simulink model "asbCubeSatACS"  (R2023b)
settings: Solver=FixedStepDiscrete  StartTime=0.0  StopTime=10.0  FixedStep=CubeSatTimeStep  RelTol=1e-3  EnableMultiTasking=on
settings Model: DataDictionary=asbCubeSatModelData.sldd  Creator=The MathWorks, Inc.  LastModifiedBy=bobow
settings SolverCC: AlgebraicLoopSolver=TrustRegion  MaxZcPerStep=1
settings DataIOCC: LimitDataPoints=on  SaveFormat=Array  SaveOutput=off  SignalLogging=off  DSMLogging=off  SaveTime=off  ReturnWorkspaceOutputs=off
settings OptimizationCC: DefaultParameterBehavior=Inlined  OptimizeBlockIOStorage=off  BufferReuse=off  GlobalBufferReuse=off  ExpressionFolding=off  ExpressionDepthLimit=2147483647  LocalBlockOutputs=off  InitFltsAndDblsToZero=on  LifeSpan=inf  OptimizeDataStoreBuffers=off  BusAssignmentInplaceUpdate=off
settings DebuggingCC: ArtificialAlgebraicLoopMsg=none  SolverPrmCheckMsg=warning  FcnCallInpInsideContextMsg=warning  UnconnectedInputMsg=warning  UnconnectedOutputMsg=warning  UnconnectedLineMsg=warning  StateNameClashWarn=warning  PregeneratedLibrarySubsystemCodeDiagnostic=none  SFUnexpectedBacktrackingDiag=warning  SFNoUnconditionalDefaultTransitionDiag=warning  SFExecutionAtInitializationDiag=none  ArithmeticOperatorsInVariantConditions=warning
settings HardwareCC: ProdBitPerPointer=32  ProdBitPerSizeT=32  ProdBitPerPtrDiffT=32  ProdLargestAtomicFloat=None  ProdIntDivRoundTo=Undefined  ProdEndianess=Unspecified  ProdWordSize=32  ProdHWDeviceType=32-bit Generic
settings ModelReferenceCC: EnableRefExpFcnMdlSchedulingChecks=on  PropagateSignalLabelsOutOfModel=off
settings SFSimCC: SimUseLocalCustomCode=off
settings RTWCC: RTWUseLocalCustomCode=off  DLArmComputeVersion=19.05
settings CodeAppCC: StateflowObjectComments=on
settings GRTTargetCC: TargetFcnLib=ansi_tfl_tmw.mat  TargetLangStandard=C89/C90 (ANSI)  CombineOutputUpdateFcns=off  GRTInterface=on
settings ConfigComp: CovMetricSettings=dw  CovSaveCumulativeToWorkspaceVar=on  CovSaveSingleToWorkspaceVar=on  CovExternalEMLEnable=off

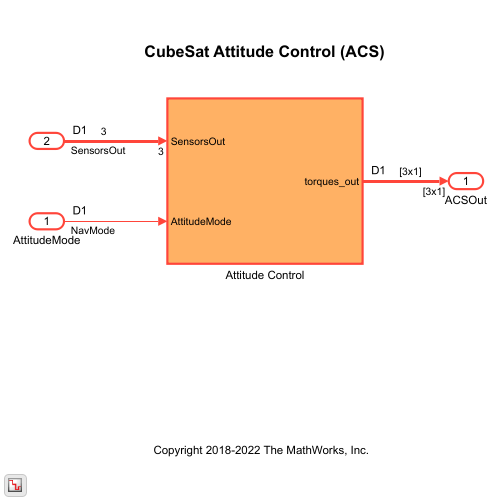
[thumbnail: Simulink's stored preview of the top-level diagram]
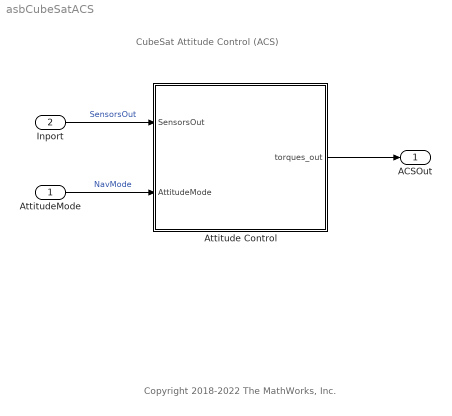
== system asbCubeSatACS ==
  note: Copyright 2018-2022 The MathWorks, Inc.
  note: CubeSat Attitude Control (ACS)
  AttitudeMode : Inport  OutDataTypeStr=double  PortDimensions=1
  Inport : Inport  Port=2  OutDataTypeStr=double
  Attitude Control : Subsystem
  ACSOut : Outport  VectorParamsAs1DForOutWhenUnconnected=off  BusOutputAsStruct=on
  wires:
  AttitudeMode/1 -> Attitude Control/2("AttitudeMode ")  "NavMode"
  Inport/1 -> Attitude Control/1(SensorsOut)  "SensorsOut"
  Attitude Control/1(torques_out) -> ACSOut/1

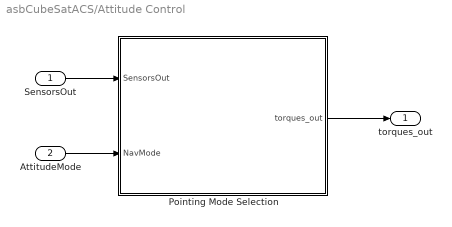
== system asbCubeSatACS/Attitude Control ==
  SensorsOut : Inport
  "AttitudeMode " : Inport  Port=2
  Pointing Mode Selection : Stateflow chart  RequirementInfo="{}  %GIDa_a065c7c8_537d_4123_b3cc_6e7e7008a32c"  TreatAsAtomicUnit=on
  torques_out : Outport  VectorParamsAs1DForOutWhenUnconnected=off
  wires:
  "AttitudeMode "/1 -> Pointing Mode Selection/2(NavMode)
  Pointing Mode Selection/1(torques_out) -> torques_out/1
  SensorsOut/1 -> Pointing Mode Selection/1(SensorsOut)

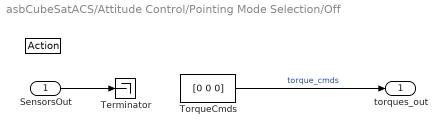
== system asbCubeSatACS/Attitude Control/Pointing Mode Selection/Off ==
  SensorsOut : Inport
  " " : ActionPort
      settings: CopyFcn=Stateflow.SLINSF.SimulinkMan.removeBlockPreDeleteFcn  PreDeleteFcn=Stateflow.SLINSF.SimulinkMan.unsafePredeleteFcn
  Terminator : Terminator
  TorqueCmds : Constant  Value=[0 0 0]
  torques_out : Outport  RequirementInfo="{}  %GIDa_4dc055f9_6cac_42e1_8ddb_4145586b89f5"  VectorParamsAs1DForOutWhenUnconnected=off
  wires:
  TorqueCmds/1 -> torques_out/1  "torque_cmds"
  SensorsOut/1 -> Terminator/1

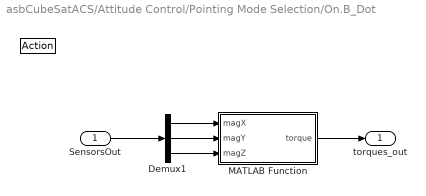
== system asbCubeSatACS/Attitude Control/Pointing Mode Selection/On.B_Dot ==
  SensorsOut : Inport
  " " : ActionPort
      settings: CopyFcn=Stateflow.SLINSF.SimulinkMan.removeBlockPreDeleteFcn  PreDeleteFcn=Stateflow.SLINSF.SimulinkMan.unsafePredeleteFcn
  Demux1 : Demux  Outputs=3
  MATLAB Function : MATLAB Function  TreatAsAtomicUnit=on
  torques_out : Outport  VectorParamsAs1DForOutWhenUnconnected=off
  wires:
  Demux1/2 -> MATLAB Function/2(magY)
  Demux1/3 -> MATLAB Function/3(magZ)
  Demux1/1 -> MATLAB Function/1(magX)
  MATLAB Function/1(torque) -> torques_out/1
  SensorsOut/1 -> Demux1/1

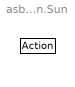
== system asbCubeSatACS/Attitude Control/Pointing Mode Selection/On.Sun ==
  " " : ActionPort
      settings: CopyFcn=Stateflow.SLINSF.SimulinkMan.removeBlockPreDeleteFcn  PreDeleteFcn=Stateflow.SLINSF.SimulinkMan.unsafePredeleteFcn

== stateflow chart asbCubeSatACS/Attitude Control/Pointing Mode Selection ==
  state On
    state Transition
    state B_Dot
    state Sun [commented out]
    (default) -> Transition
    Transition -> Sun [commented out] : [NavMode == 2]
    Sun -> Transition [commented out] : [NavMode == 1]
    Transition -> B_Dot : [NavMode == 1]
    B_Dot -> Transition : [NavMode == 2]
  state Off
  (default) -> Off
  Off -> On : [NavMode ~= 0]
  On -> Off : [NavMode == 0]
  data: sf_internal_action_state_placeholder_data local double size=1 =0; sf_internal_action_state_placeholder_data local double size=1 =0; sf_internal_action_state_placeholder_data local double size=1 =0; SensorsOut input; NavMode input; torques_out output =[0 0 0]'

== matlab function asbCubeSatACS/Attitude Control/Pointing Mode Selection/On.B_Dot/MATLAB Function ==
  data: torque output; magX input; magY input; magZ input
function torque = fcn(magX, magY, magZ)
    persistent coreMagX coreMagY airMagZ prev_measurement
    % Define the parameters
    core_radius = 0.005;
    core_length = 0.045;
    layers = 6;
    temp = 20;
    side_length = 0.045;
    air_length = 0.025;
    air_layers = 5; 

    if isempty(coreMagX) || isempty(coreMagY) || isempty(airMagZ)
        coreMagX = CoreMagnetorquer(core_radius, core_length, layers, temp);
        coreMagY = CoreMagnetorquer(core_radius, core_length, layers, temp);  
        airMagZ = AirMagnetorquer(side_length, air_length, air_layers, temp);
    end

    magnetometer_measurements = [magX; magY; magZ];

    if isempty(prev_measurement)
        prev_measurement = magnetometer_measurements;
    end

    b_dot = (magnetometer_measurements - prev_measurement);
    
    m = -b_dot * 1e9;
   
    if abs(m(1)) > coreMagX.max_dipole
        m = m .* coreMagX.max_dipole ./ abs(m(1));
    end
    if abs(m(2)) > coreMagY.max_dipole
        m = m .* coreMagY.max_dipole ./ abs(m(2));
    end
    if abs(m(3)) > airMagZ.max_dipole
        m = m .* airMagZ.max_dipole ./ abs(m(3));
    end
    prev_measurement = magnetometer_measurements;

    % Torque = m x B
    torque = cross(m, magnetometer_measurements);
